simulink model "untitled"  (R2019b)
settings: Solver=VariableStepAuto  StartTime=0.0  StopTime=10.0  RelTol=1e-3
values from neighbouring files (symbols this model uses):
  C = 1    [DataLoop.m]    (also in run_iso_calc.m; testLoop.m = 1.2)
  t_current = 0    [DataLoop.m]    (also in run_iso_calc.m = t; testLoop.m)
  Tr = 1    [DataLoop.m]    (also in run_iso_calc.m = 0.38; testLoop.m = 0.38)
  Ts = 1    [DataLoop.m]    (also in run_iso_calc.m = 0.5; testLoop.m = 0.5)
  Vh = rand    [run_iso_calc.m]
  Vs = 1    [DataLoop.m]    (also in run_iso_calc.m = rand; testLoop.m = 0)
  Zd = 1    [DataLoop.m]    (also in run_iso_calc.m = 0.02; testLoop.m = 0.02)
  Zr = 1    [DataLoop.m]    (also in run_iso_calc.m = 0; testLoop.m = 0)
settings Model: Creator=laiy  LastModifiedBy=laiy

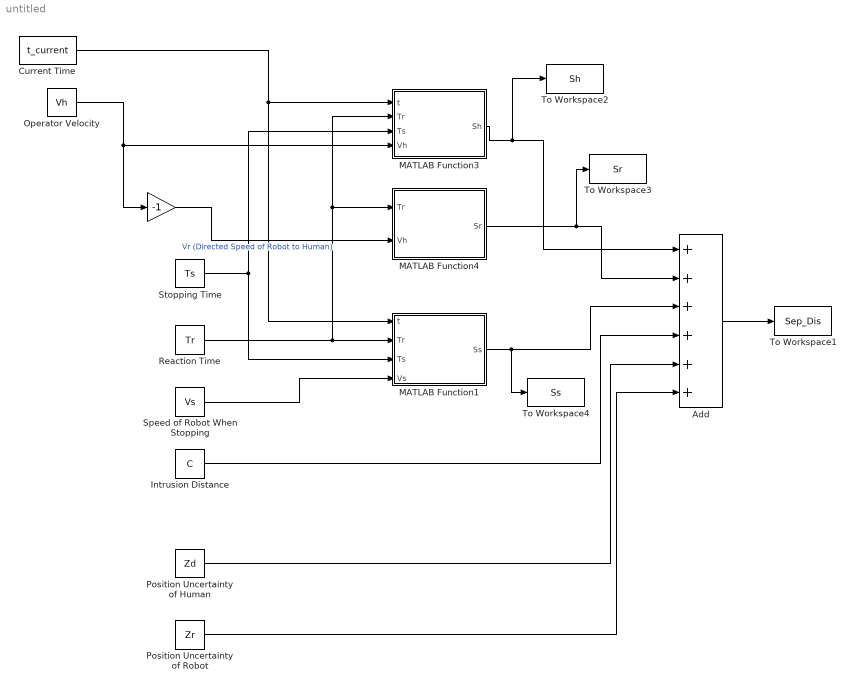
== system untitled ==
  " " : Gain  Gain=-1
  Add : Sum  Inputs=++++++
  Current Time : Constant  Value=t_current
  Intrusion Distance : Constant  Value=C
  MATLAB Function1 : MATLAB Function  TreatAsAtomicUnit=on
  MATLAB Function3 : MATLAB Function  TreatAsAtomicUnit=on
  MATLAB Function4 : MATLAB Function  TreatAsAtomicUnit=on
  Operator Velocity : Constant  Value=Vh
  Position Uncertainty of Human : Constant  Value=Zd
  Position Uncertainty of Robot : Constant  Value=Zr
  Reaction Time : Constant  Value=Tr
  Speed of Robot When Stopping : Constant  Value=Vs
  Stopping Time : Constant  Value=Ts
  To Workspace1 : ToWorkspace  VariableName=Sep_Dis  SampleTime=-1
  To Workspace2 : ToWorkspace  VariableName=Sh  SampleTime=-1
  To Workspace3 : ToWorkspace  VariableName=Sr  SampleTime=-1
  To Workspace4 : ToWorkspace  VariableName=Ss  SampleTime=-1
  wires:
  Current Time/1 -> MATLAB Function1/1(t), MATLAB Function3/1(t)
  MATLAB Function4/1(Sr) -> To Workspace3/1, Add/2
  MATLAB Function1/1(Ss) -> To Workspace4/1, Add/3
  MATLAB Function3/1(Sh) -> To Workspace2/1, Add/1
  Position Uncertainty of Human/1 -> Add/5
  Reaction Time/1 -> MATLAB Function1/2(Tr), MATLAB Function4/1(Tr), MATLAB Function3/2(Tr)
  Operator Velocity/1 -> MATLAB Function3/4(Vh), " "/1
  " "/1 -> MATLAB Function4/2(Vh)  "Vr (Directed Speed of Robot to Human)"
  Position Uncertainty of Robot/1 -> Add/6
  Stopping Time/1 -> MATLAB Function3/3(Ts), MATLAB Function1/3(Ts)
  Intrusion Distance/1 -> Add/4
  Speed of Robot When Stopping/1 -> MATLAB Function1/4(Vs)
  Add/1 -> To Workspace1/1

== matlab function untitled/MATLAB Function4 ==
  data: Tr input; Vh input; Sr output
function Sr = fcn(Tr, Vh)

% separation distance due to robot motion
% Vr is assumed to reduces the separation distance the most

Sr = Tr * Vh;

== matlab function untitled/MATLAB Function3 ==
  data: t input; Sh output; Tr input; Ts input; Vh input
function Sh = fcn(t, Tr, Ts, Vh)

% separation distance due to operator's change in location

t_int = t:0.001:t+Tr+Ts;
v = zeros(length(t_int),1) + Vh;

Sh = trapz(t_int,v);

== matlab function untitled/MATLAB Function1 ==
  data: t input; Tr input; Ss output; Ts input; Vs input
function Ss = fcn(t, Tr, Ts, Vs)

% separation distance due to robot stopping

t_int = t+Tr:0.001:t+Tr+Ts;
v = zeros(length(t_int),1) + Vs;

Ss = trapz(t_int,v);
